simulink model "VSD_FD_codegen_V2"  (R2021b)
settings: Solver=FixedStepDiscrete  StartTime=0.0  StopTime=2  RelTol=1e-3  EnableMultiTasking=on
PreLoadFcn:
  | uz_setCodegenPaths
model workspace (MATLAB code in the model file):
  | cmdLim = Simulink.Parameter;
  | cmdLim.Value = 15;
  | cmdLim.Description = 'Limit for controlling the maximum surface command angle.';
  | cmdLim.Min = 0;
  | cmdLim.Max = 90;
  | cmdLim.DocUnits = 'deg';
  | 
  | dispGain = Simulink.Parameter;
  | dispGain.Value = 0.75;
  | dispGain.Description = 'Gain applied to the displacement error.';
  | dispGain.Min = 0;
  | dispGain.Max = [];
  | dispGain.DocUnits = 'deg/sec/deg';
  | 
  | dispLim = Simulink.Parameter;
  | dispLim.Value = 30;
  | dispLim.Description = 'Limit for controlling the maximum commanded angle.';
  | dispLim.Min = 0;
  | dispLim.Max = 180;
  | dispLim.DocUnits = 'deg';
  | 
  | intGain = Simulink.Parameter;
  | intGain.Value = 0.5;
  | intGain.Description = 'Gain applied to the integral error.';
  | intGain.Min = 0;
  | intGain.Max = [];
  | intGain.DocUnits = 'deg/sec/deg/sec';
  | 
  | intLim = Simulink.Parameter;
  | intLim.Value = 5;
  | intLim.Description = 'Limit for controlling the maximum commanded angle.';
  | intLim.Min = 0;
  | intLim.Max = 90;
  | intLim.DocUnits = 'deg';
  | 
  | rateGain = Simulink.Parameter;
  | rateGain.Value = 2;
  | rateGain.Description = 'Gain applied to the rate error.';
  | rateGain.Min = 0;
  | rateGain.Max = [];
  | rateGain.DocUnits = 'deg/deg/sec';
  | 
  | rateLim = Simulink.Parameter;
  | rateLim.Value = 6;
  | rateLim.Description = 'Limit for controlling the maximum commanded angle.';
  | rateLim.Min = 0;
  | rateLim.Max = 180;
  | rateLim.DocUnits = 'deg/sec';
  | 
  | hdgGain = Simulink.Parameter;
  | hdgGain.Value = 0.015;
undefined symbols (not defined in the file or in its folder): DiscIntNeverNeededParam, f_FD
libraries: simulink x203, dspstat3 x3, spsFirstOrderFilterLib x2
(part 2 of 2)

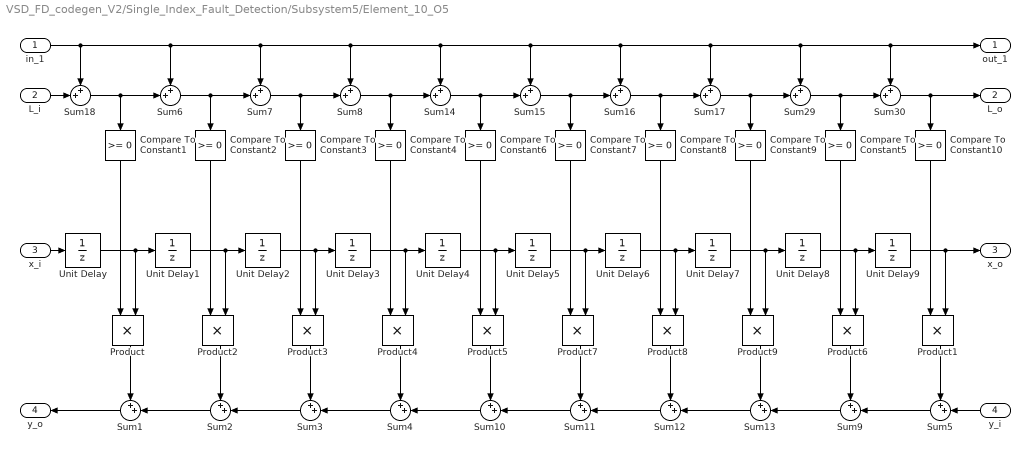
== system VSD_FD_codegen_V2/Single_Index_Fault_Detection/Subsystem5/Element_10_O5 ==
  in_1 : Inport
  L_i : Inport  Port=2
  x_i : Inport  Port=3
  y_i : Inport  Port=4
  Compare To Constant{1..10} (10 alike) : simulink/Logic and Bit Operations/Compare To Constant  relop=>=  const=0  OutDataTypeStr=boolean
  Product{,1..9} (10 alike) : Product
  Sum{1..18,29..30} (20 alike) : Sum  Inputs=++|
  Unit Delay{,1..9} (10 alike) : UnitDelay  SampleTime=-1  HasFrameUpgradeWarning=on
  out_1 : Outport
  L_o : Outport  Port=2
  x_o : Outport  Port=3
  y_o : Outport  Port=4
  wires:
  Sum2/1 -> Sum1/2
  Unit Delay4/1 -> Unit Delay5/1, Product5/2
  Unit Delay9/1 -> x_o/1, Product1/2
  Sum3/1 -> Sum2/2
  Sum6/1 -> Compare To Constant2/1, Sum7/2
  Sum15/1 -> Compare To Constant7/1, Sum16/2
  Sum9/1 -> Sum13/2
  Sum14/1 -> Sum15/2, Compare To Constant6/1
  Compare To Constant4/1 -> Product4/1
  Unit Delay7/1 -> Unit Delay8/1, Product9/2
  Unit Delay6/1 -> Unit Delay7/1, Product8/2
  Sum7/1 -> Compare To Constant3/1, Sum8/2
  Compare To Constant3/1 -> Product3/1
  Product8/1 -> Sum12/1
  Sum13/1 -> Sum12/2
  in_1/1 -> Sum18/1, Sum6/1, Sum7/1, Sum15/1, Sum16/1, out_1/1, Sum30/1, Sum29/1, Sum17/1, Sum14/1, Sum8/1
  Unit Delay8/1 -> Unit Delay9/1, Product6/2
  Product9/1 -> Sum13/1
  Sum11/1 -> Sum10/2
  Sum8/1 -> Compare To Constant4/1, Sum14/2
  Compare To Constant6/1 -> Product5/1
  Product7/1 -> Sum11/1
  Compare To Constant8/1 -> Product8/1
  Product/1 -> Sum1/1
  Unit Delay5/1 -> Unit Delay6/1, Product7/2
  Unit Delay/1 -> Unit Delay1/1, Product/2
  Unit Delay1/1 -> Unit Delay2/1, Product2/2
  Compare To Constant5/1 -> Product6/1
  Sum10/1 -> Sum4/2
  Sum1/1 -> y_o/1
  Compare To Constant2/1 -> Product2/1
  Sum16/1 -> Compare To Constant8/1, Sum17/2
  Compare To Constant1/1 -> Product/1
  Sum4/1 -> Sum3/2
  Sum17/1 -> Sum29/2, Compare To Constant9/1
  Unit Delay3/1 -> Unit Delay4/1, Product4/2
  Product5/1 -> Sum10/1
  Product6/1 -> Sum9/1
  Sum12/1 -> Sum11/2
  Sum29/1 -> Sum30/2, Compare To Constant5/1
  Sum30/1 -> L_o/1, Compare To Constant10/1
  Product4/1 -> Sum4/1
  Product2/1 -> Sum2/1
  Unit Delay2/1 -> Unit Delay3/1, Product3/2
  Compare To Constant9/1 -> Product9/1
  Product3/1 -> Sum3/1
  x_i/1 -> Unit Delay/1
  Compare To Constant7/1 -> Product7/1
  Compare To Constant10/1 -> Product1/1
  Product1/1 -> Sum5/1
  y_i/1 -> Sum5/2
  Sum5/1 -> Sum9/2
  L_i/1 -> Sum18/2
  Sum18/1 -> Compare To Constant1/1, Sum6/2

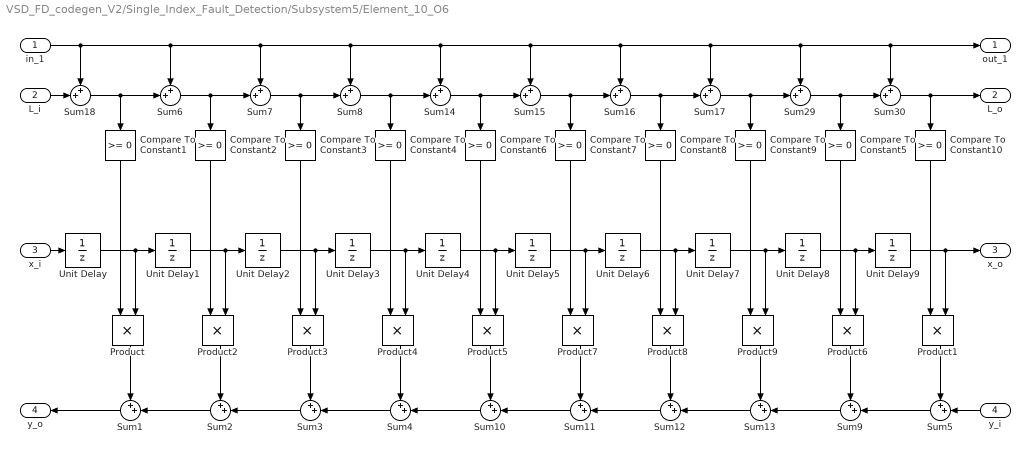
== system VSD_FD_codegen_V2/Single_Index_Fault_Detection/Subsystem5/Element_10_O6 ==
  in_1 : Inport
  L_i : Inport  Port=2
  x_i : Inport  Port=3
  y_i : Inport  Port=4
  Compare To Constant{1..10} (10 alike) : simulink/Logic and Bit Operations/Compare To Constant  relop=>=  const=0  OutDataTypeStr=boolean
  Product{,1..9} (10 alike) : Product
  Sum{1..18,29..30} (20 alike) : Sum  Inputs=++|
  Unit Delay{,1..9} (10 alike) : UnitDelay  SampleTime=-1  HasFrameUpgradeWarning=on
  out_1 : Outport
  L_o : Outport  Port=2
  x_o : Outport  Port=3
  y_o : Outport  Port=4
  wires:
  Sum2/1 -> Sum1/2
  Unit Delay4/1 -> Unit Delay5/1, Product5/2
  Unit Delay9/1 -> x_o/1, Product1/2
  Sum3/1 -> Sum2/2
  Sum6/1 -> Compare To Constant2/1, Sum7/2
  Sum15/1 -> Compare To Constant7/1, Sum16/2
  Sum9/1 -> Sum13/2
  Sum14/1 -> Sum15/2, Compare To Constant6/1
  Compare To Constant4/1 -> Product4/1
  Unit Delay7/1 -> Unit Delay8/1, Product9/2
  Unit Delay6/1 -> Unit Delay7/1, Product8/2
  Sum7/1 -> Compare To Constant3/1, Sum8/2
  Compare To Constant3/1 -> Product3/1
  Product8/1 -> Sum12/1
  Sum13/1 -> Sum12/2
  in_1/1 -> Sum18/1, Sum6/1, Sum7/1, Sum15/1, Sum16/1, out_1/1, Sum30/1, Sum29/1, Sum17/1, Sum14/1, Sum8/1
  Unit Delay8/1 -> Unit Delay9/1, Product6/2
  Product9/1 -> Sum13/1
  Sum11/1 -> Sum10/2
  Sum8/1 -> Compare To Constant4/1, Sum14/2
  Compare To Constant6/1 -> Product5/1
  Product7/1 -> Sum11/1
  Compare To Constant8/1 -> Product8/1
  Product/1 -> Sum1/1
  Unit Delay5/1 -> Unit Delay6/1, Product7/2
  Unit Delay/1 -> Unit Delay1/1, Product/2
  Unit Delay1/1 -> Unit Delay2/1, Product2/2
  Compare To Constant5/1 -> Product6/1
  Sum10/1 -> Sum4/2
  Sum1/1 -> y_o/1
  Compare To Constant2/1 -> Product2/1
  Sum16/1 -> Compare To Constant8/1, Sum17/2
  Compare To Constant1/1 -> Product/1
  Sum4/1 -> Sum3/2
  Sum17/1 -> Sum29/2, Compare To Constant9/1
  Unit Delay3/1 -> Unit Delay4/1, Product4/2
  Product5/1 -> Sum10/1
  Product6/1 -> Sum9/1
  Sum12/1 -> Sum11/2
  Sum29/1 -> Sum30/2, Compare To Constant5/1
  Sum30/1 -> L_o/1, Compare To Constant10/1
  Product4/1 -> Sum4/1
  Product2/1 -> Sum2/1
  Unit Delay2/1 -> Unit Delay3/1, Product3/2
  Compare To Constant9/1 -> Product9/1
  Product3/1 -> Sum3/1
  x_i/1 -> Unit Delay/1
  Compare To Constant7/1 -> Product7/1
  Compare To Constant10/1 -> Product1/1
  Product1/1 -> Sum5/1
  y_i/1 -> Sum5/2
  Sum5/1 -> Sum9/2
  L_i/1 -> Sum18/2
  Sum18/1 -> Compare To Constant1/1, Sum6/2

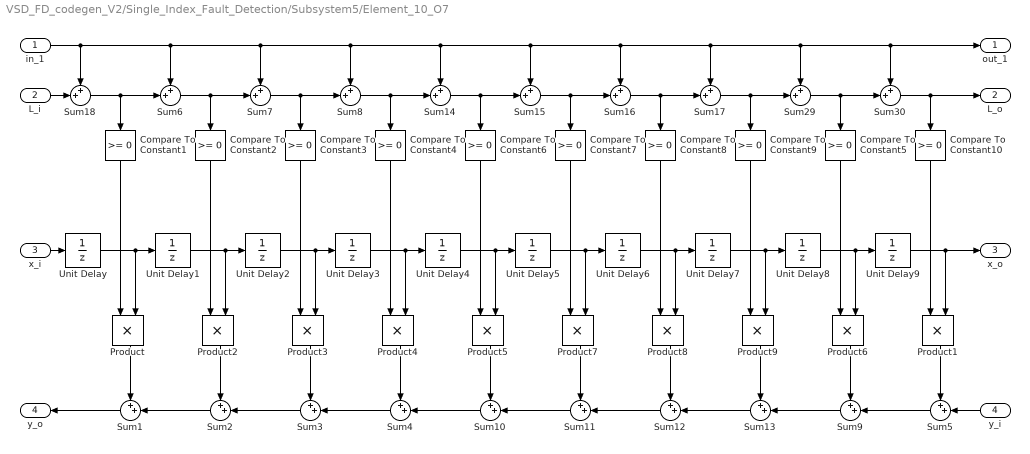
== system VSD_FD_codegen_V2/Single_Index_Fault_Detection/Subsystem5/Element_10_O7 ==
  in_1 : Inport
  L_i : Inport  Port=2
  x_i : Inport  Port=3
  y_i : Inport  Port=4
  Compare To Constant{1..10} (10 alike) : simulink/Logic and Bit Operations/Compare To Constant  relop=>=  const=0  OutDataTypeStr=boolean
  Product{,1..9} (10 alike) : Product
  Sum{1..18,29..30} (20 alike) : Sum  Inputs=++|
  Unit Delay{,1..9} (10 alike) : UnitDelay  SampleTime=-1  HasFrameUpgradeWarning=on
  out_1 : Outport
  L_o : Outport  Port=2
  x_o : Outport  Port=3
  y_o : Outport  Port=4
  wires:
  Sum2/1 -> Sum1/2
  Unit Delay4/1 -> Unit Delay5/1, Product5/2
  Unit Delay9/1 -> x_o/1, Product1/2
  Sum3/1 -> Sum2/2
  Sum6/1 -> Compare To Constant2/1, Sum7/2
  Sum15/1 -> Compare To Constant7/1, Sum16/2
  Sum9/1 -> Sum13/2
  Sum14/1 -> Sum15/2, Compare To Constant6/1
  Compare To Constant4/1 -> Product4/1
  Unit Delay7/1 -> Unit Delay8/1, Product9/2
  Unit Delay6/1 -> Unit Delay7/1, Product8/2
  Sum7/1 -> Compare To Constant3/1, Sum8/2
  Compare To Constant3/1 -> Product3/1
  Product8/1 -> Sum12/1
  Sum13/1 -> Sum12/2
  in_1/1 -> Sum18/1, Sum6/1, Sum7/1, Sum15/1, Sum16/1, out_1/1, Sum30/1, Sum29/1, Sum17/1, Sum14/1, Sum8/1
  Unit Delay8/1 -> Unit Delay9/1, Product6/2
  Product9/1 -> Sum13/1
  Sum11/1 -> Sum10/2
  Sum8/1 -> Compare To Constant4/1, Sum14/2
  Compare To Constant6/1 -> Product5/1
  Product7/1 -> Sum11/1
  Compare To Constant8/1 -> Product8/1
  Product/1 -> Sum1/1
  Unit Delay5/1 -> Unit Delay6/1, Product7/2
  Unit Delay/1 -> Unit Delay1/1, Product/2
  Unit Delay1/1 -> Unit Delay2/1, Product2/2
  Compare To Constant5/1 -> Product6/1
  Sum10/1 -> Sum4/2
  Sum1/1 -> y_o/1
  Compare To Constant2/1 -> Product2/1
  Sum16/1 -> Compare To Constant8/1, Sum17/2
  Compare To Constant1/1 -> Product/1
  Sum4/1 -> Sum3/2
  Sum17/1 -> Sum29/2, Compare To Constant9/1
  Unit Delay3/1 -> Unit Delay4/1, Product4/2
  Product5/1 -> Sum10/1
  Product6/1 -> Sum9/1
  Sum12/1 -> Sum11/2
  Sum29/1 -> Sum30/2, Compare To Constant5/1
  Sum30/1 -> L_o/1, Compare To Constant10/1
  Product4/1 -> Sum4/1
  Product2/1 -> Sum2/1
  Unit Delay2/1 -> Unit Delay3/1, Product3/2
  Compare To Constant9/1 -> Product9/1
  Product3/1 -> Sum3/1
  x_i/1 -> Unit Delay/1
  Compare To Constant7/1 -> Product7/1
  Compare To Constant10/1 -> Product1/1
  Product1/1 -> Sum5/1
  y_i/1 -> Sum5/2
  Sum5/1 -> Sum9/2
  L_i/1 -> Sum18/2
  Sum18/1 -> Compare To Constant1/1, Sum6/2

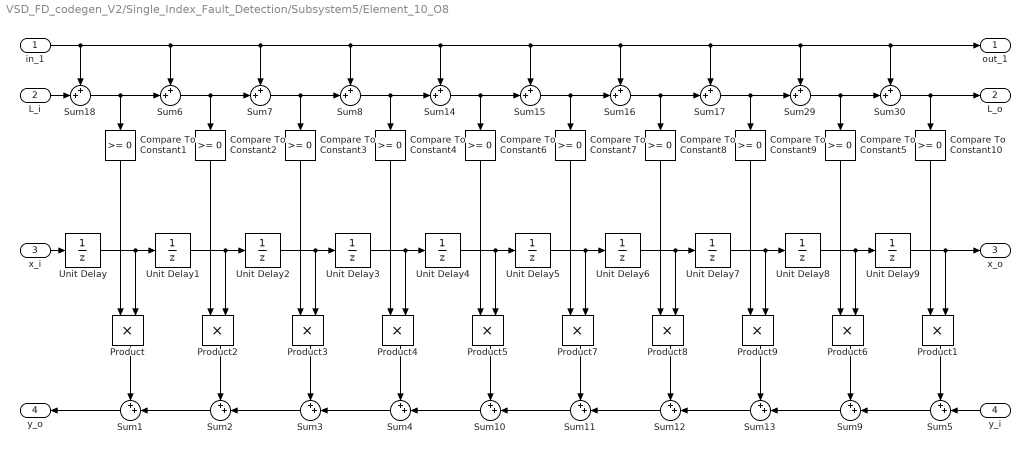
== system VSD_FD_codegen_V2/Single_Index_Fault_Detection/Subsystem5/Element_10_O8 ==
  in_1 : Inport
  L_i : Inport  Port=2
  x_i : Inport  Port=3
  y_i : Inport  Port=4
  Compare To Constant{1..10} (10 alike) : simulink/Logic and Bit Operations/Compare To Constant  relop=>=  const=0  OutDataTypeStr=boolean
  Product{,1..9} (10 alike) : Product
  Sum{1..18,29..30} (20 alike) : Sum  Inputs=++|
  Unit Delay{,1..9} (10 alike) : UnitDelay  SampleTime=-1  HasFrameUpgradeWarning=on
  out_1 : Outport
  L_o : Outport  Port=2
  x_o : Outport  Port=3
  y_o : Outport  Port=4
  wires:
  Sum2/1 -> Sum1/2
  Unit Delay4/1 -> Unit Delay5/1, Product5/2
  Unit Delay9/1 -> x_o/1, Product1/2
  Sum3/1 -> Sum2/2
  Sum6/1 -> Compare To Constant2/1, Sum7/2
  Sum15/1 -> Compare To Constant7/1, Sum16/2
  Sum9/1 -> Sum13/2
  Sum14/1 -> Sum15/2, Compare To Constant6/1
  Compare To Constant4/1 -> Product4/1
  Unit Delay7/1 -> Unit Delay8/1, Product9/2
  Unit Delay6/1 -> Unit Delay7/1, Product8/2
  Sum7/1 -> Compare To Constant3/1, Sum8/2
  Compare To Constant3/1 -> Product3/1
  Product8/1 -> Sum12/1
  Sum13/1 -> Sum12/2
  in_1/1 -> Sum18/1, Sum6/1, Sum7/1, Sum15/1, Sum16/1, out_1/1, Sum30/1, Sum29/1, Sum17/1, Sum14/1, Sum8/1
  Unit Delay8/1 -> Unit Delay9/1, Product6/2
  Product9/1 -> Sum13/1
  Sum11/1 -> Sum10/2
  Sum8/1 -> Compare To Constant4/1, Sum14/2
  Compare To Constant6/1 -> Product5/1
  Product7/1 -> Sum11/1
  Compare To Constant8/1 -> Product8/1
  Product/1 -> Sum1/1
  Unit Delay5/1 -> Unit Delay6/1, Product7/2
  Unit Delay/1 -> Unit Delay1/1, Product/2
  Unit Delay1/1 -> Unit Delay2/1, Product2/2
  Compare To Constant5/1 -> Product6/1
  Sum10/1 -> Sum4/2
  Sum1/1 -> y_o/1
  Compare To Constant2/1 -> Product2/1
  Sum16/1 -> Compare To Constant8/1, Sum17/2
  Compare To Constant1/1 -> Product/1
  Sum4/1 -> Sum3/2
  Sum17/1 -> Sum29/2, Compare To Constant9/1
  Unit Delay3/1 -> Unit Delay4/1, Product4/2
  Product5/1 -> Sum10/1
  Product6/1 -> Sum9/1
  Sum12/1 -> Sum11/2
  Sum29/1 -> Sum30/2, Compare To Constant5/1
  Sum30/1 -> L_o/1, Compare To Constant10/1
  Product4/1 -> Sum4/1
  Product2/1 -> Sum2/1
  Unit Delay2/1 -> Unit Delay3/1, Product3/2
  Compare To Constant9/1 -> Product9/1
  Product3/1 -> Sum3/1
  x_i/1 -> Unit Delay/1
  Compare To Constant7/1 -> Product7/1
  Compare To Constant10/1 -> Product1/1
  Product1/1 -> Sum5/1
  y_i/1 -> Sum5/2
  Sum5/1 -> Sum9/2
  L_i/1 -> Sum18/2
  Sum18/1 -> Compare To Constant1/1, Sum6/2

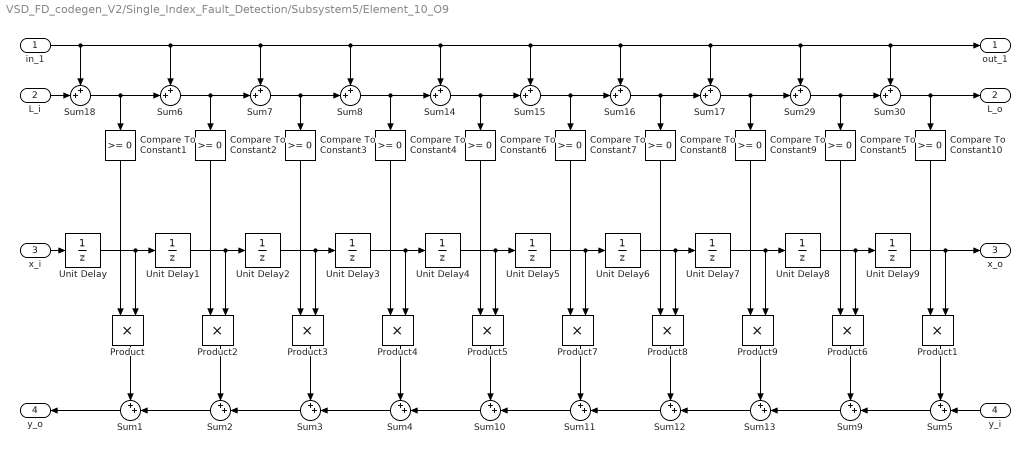
== system VSD_FD_codegen_V2/Single_Index_Fault_Detection/Subsystem5/Element_10_O9 ==
  in_1 : Inport
  L_i : Inport  Port=2
  x_i : Inport  Port=3
  y_i : Inport  Port=4
  Compare To Constant{1..10} (10 alike) : simulink/Logic and Bit Operations/Compare To Constant  relop=>=  const=0  OutDataTypeStr=boolean
  Product{,1..9} (10 alike) : Product
  Sum{1..18,29..30} (20 alike) : Sum  Inputs=++|
  Unit Delay{,1..9} (10 alike) : UnitDelay  SampleTime=-1  HasFrameUpgradeWarning=on
  out_1 : Outport
  L_o : Outport  Port=2
  x_o : Outport  Port=3
  y_o : Outport  Port=4
  wires:
  Sum2/1 -> Sum1/2
  Unit Delay4/1 -> Unit Delay5/1, Product5/2
  Unit Delay9/1 -> x_o/1, Product1/2
  Sum3/1 -> Sum2/2
  Sum6/1 -> Compare To Constant2/1, Sum7/2
  Sum15/1 -> Compare To Constant7/1, Sum16/2
  Sum9/1 -> Sum13/2
  Sum14/1 -> Sum15/2, Compare To Constant6/1
  Compare To Constant4/1 -> Product4/1
  Unit Delay7/1 -> Unit Delay8/1, Product9/2
  Unit Delay6/1 -> Unit Delay7/1, Product8/2
  Sum7/1 -> Compare To Constant3/1, Sum8/2
  Compare To Constant3/1 -> Product3/1
  Product8/1 -> Sum12/1
  Sum13/1 -> Sum12/2
  in_1/1 -> Sum18/1, Sum6/1, Sum7/1, Sum15/1, Sum16/1, out_1/1, Sum30/1, Sum29/1, Sum17/1, Sum14/1, Sum8/1
  Unit Delay8/1 -> Unit Delay9/1, Product6/2
  Product9/1 -> Sum13/1
  Sum11/1 -> Sum10/2
  Sum8/1 -> Compare To Constant4/1, Sum14/2
  Compare To Constant6/1 -> Product5/1
  Product7/1 -> Sum11/1
  Compare To Constant8/1 -> Product8/1
  Product/1 -> Sum1/1
  Unit Delay5/1 -> Unit Delay6/1, Product7/2
  Unit Delay/1 -> Unit Delay1/1, Product/2
  Unit Delay1/1 -> Unit Delay2/1, Product2/2
  Compare To Constant5/1 -> Product6/1
  Sum10/1 -> Sum4/2
  Sum1/1 -> y_o/1
  Compare To Constant2/1 -> Product2/1
  Sum16/1 -> Compare To Constant8/1, Sum17/2
  Compare To Constant1/1 -> Product/1
  Sum4/1 -> Sum3/2
  Sum17/1 -> Sum29/2, Compare To Constant9/1
  Unit Delay3/1 -> Unit Delay4/1, Product4/2
  Product5/1 -> Sum10/1
  Product6/1 -> Sum9/1
  Sum12/1 -> Sum11/2
  Sum29/1 -> Sum30/2, Compare To Constant5/1
  Sum30/1 -> L_o/1, Compare To Constant10/1
  Product4/1 -> Sum4/1
  Product2/1 -> Sum2/1
  Unit Delay2/1 -> Unit Delay3/1, Product3/2
  Compare To Constant9/1 -> Product9/1
  Product3/1 -> Sum3/1
  x_i/1 -> Unit Delay/1
  Compare To Constant7/1 -> Product7/1
  Compare To Constant10/1 -> Product1/1
  Product1/1 -> Sum5/1
  y_i/1 -> Sum5/2
  Sum5/1 -> Sum9/2
  L_i/1 -> Sum18/2
  Sum18/1 -> Compare To Constant1/1, Sum6/2

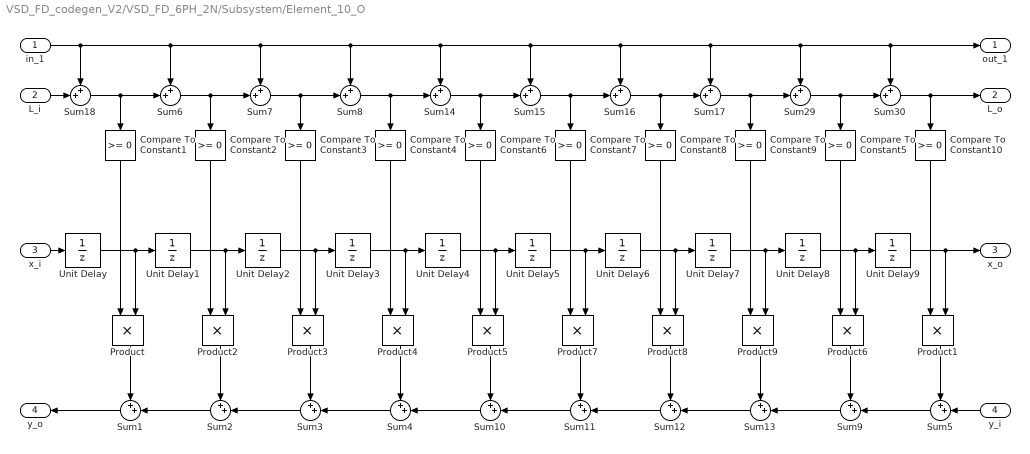
== system VSD_FD_codegen_V2/VSD_FD_6PH_2N/Subsystem/Element_10_O ==
  in_1 : Inport
  L_i : Inport  Port=2
  x_i : Inport  Port=3
  y_i : Inport  Port=4
  Compare To Constant{1..10} (10 alike) : simulink/Logic and Bit Operations/Compare To Constant  relop=>=  const=0  OutDataTypeStr=boolean
  Product{,1..9} (10 alike) : Product
  Sum{1..18,29..30} (20 alike) : Sum  Inputs=++|
  Unit Delay{,1..9} (10 alike) : UnitDelay  SampleTime=-1  HasFrameUpgradeWarning=on
  out_1 : Outport
  L_o : Outport  Port=2
  x_o : Outport  Port=3
  y_o : Outport  Port=4
  wires:
  Sum2/1 -> Sum1/2
  Unit Delay4/1 -> Unit Delay5/1, Product5/2
  Unit Delay9/1 -> x_o/1, Product1/2
  Sum3/1 -> Sum2/2
  Sum6/1 -> Compare To Constant2/1, Sum7/2
  Sum15/1 -> Compare To Constant7/1, Sum16/2
  Sum9/1 -> Sum13/2
  Sum14/1 -> Sum15/2, Compare To Constant6/1
  Compare To Constant4/1 -> Product4/1
  Unit Delay7/1 -> Unit Delay8/1, Product9/2
  Unit Delay6/1 -> Unit Delay7/1, Product8/2
  Sum7/1 -> Compare To Constant3/1, Sum8/2
  Compare To Constant3/1 -> Product3/1
  Product8/1 -> Sum12/1
  Sum13/1 -> Sum12/2
  in_1/1 -> Sum18/1, Sum6/1, Sum7/1, Sum15/1, Sum16/1, out_1/1, Sum30/1, Sum29/1, Sum17/1, Sum14/1, Sum8/1
  Unit Delay8/1 -> Unit Delay9/1, Product6/2
  Product9/1 -> Sum13/1
  Sum11/1 -> Sum10/2
  Sum8/1 -> Compare To Constant4/1, Sum14/2
  Compare To Constant6/1 -> Product5/1
  Product7/1 -> Sum11/1
  Compare To Constant8/1 -> Product8/1
  Product/1 -> Sum1/1
  Unit Delay5/1 -> Unit Delay6/1, Product7/2
  Unit Delay/1 -> Unit Delay1/1, Product/2
  Unit Delay1/1 -> Unit Delay2/1, Product2/2
  Compare To Constant5/1 -> Product6/1
  Sum10/1 -> Sum4/2
  Sum1/1 -> y_o/1
  Compare To Constant2/1 -> Product2/1
  Sum16/1 -> Compare To Constant8/1, Sum17/2
  Compare To Constant1/1 -> Product/1
  Sum4/1 -> Sum3/2
  Sum17/1 -> Sum29/2, Compare To Constant9/1
  Unit Delay3/1 -> Unit Delay4/1, Product4/2
  Product5/1 -> Sum10/1
  Product6/1 -> Sum9/1
  Sum12/1 -> Sum11/2
  Sum29/1 -> Sum30/2, Compare To Constant5/1
  Sum30/1 -> L_o/1, Compare To Constant10/1
  Product4/1 -> Sum4/1
  Product2/1 -> Sum2/1
  Unit Delay2/1 -> Unit Delay3/1, Product3/2
  Compare To Constant9/1 -> Product9/1
  Product3/1 -> Sum3/1
  x_i/1 -> Unit Delay/1
  Compare To Constant7/1 -> Product7/1
  Compare To Constant10/1 -> Product1/1
  Product1/1 -> Sum5/1
  y_i/1 -> Sum5/2
  Sum5/1 -> Sum9/2
  L_i/1 -> Sum18/2
  Sum18/1 -> Compare To Constant1/1, Sum6/2

== system VSD_FD_codegen_V2/VSD_FD_6PH_2N/Subsystem/Element_10_O1 ==
  in_1 : Inport
  L_i : Inport  Port=2
  x_i : Inport  Port=3
  y_i : Inport  Port=4
  Compare To Constant{1..10} (10 alike) : simulink/Logic and Bit Operations/Compare To Constant  relop=>=  const=0  OutDataTypeStr=boolean
  Product{,1..9} (10 alike) : Product
  Sum{1..18,29..30} (20 alike) : Sum  Inputs=++|
  Unit Delay{,1..9} (10 alike) : UnitDelay  SampleTime=-1  HasFrameUpgradeWarning=on
  out_1 : Outport
  L_o : Outport  Port=2
  x_o : Outport  Port=3
  y_o : Outport  Port=4
  wires:
  Sum2/1 -> Sum1/2
  Unit Delay4/1 -> Unit Delay5/1, Product5/2
  Unit Delay9/1 -> x_o/1, Product1/2
  Sum3/1 -> Sum2/2
  Sum6/1 -> Compare To Constant2/1, Sum7/2
  Sum15/1 -> Compare To Constant7/1, Sum16/2
  Sum9/1 -> Sum13/2
  Sum14/1 -> Sum15/2, Compare To Constant6/1
  Compare To Constant4/1 -> Product4/1
  Unit Delay7/1 -> Unit Delay8/1, Product9/2
  Unit Delay6/1 -> Unit Delay7/1, Product8/2
  Sum7/1 -> Compare To Constant3/1, Sum8/2
  Compare To Constant3/1 -> Product3/1
  Product8/1 -> Sum12/1
  Sum13/1 -> Sum12/2
  in_1/1 -> Sum18/1, Sum6/1, Sum7/1, Sum15/1, Sum16/1, out_1/1, Sum30/1, Sum29/1, Sum17/1, Sum14/1, Sum8/1
  Unit Delay8/1 -> Unit Delay9/1, Product6/2
  Product9/1 -> Sum13/1
  Sum11/1 -> Sum10/2
  Sum8/1 -> Compare To Constant4/1, Sum14/2
  Compare To Constant6/1 -> Product5/1
  Product7/1 -> Sum11/1
  Compare To Constant8/1 -> Product8/1
  Product/1 -> Sum1/1
  Unit Delay5/1 -> Unit Delay6/1, Product7/2
  Unit Delay/1 -> Unit Delay1/1, Product/2
  Unit Delay1/1 -> Unit Delay2/1, Product2/2
  Compare To Constant5/1 -> Product6/1
  Sum10/1 -> Sum4/2
  Sum1/1 -> y_o/1
  Compare To Constant2/1 -> Product2/1
  Sum16/1 -> Compare To Constant8/1, Sum17/2
  Compare To Constant1/1 -> Product/1
  Sum4/1 -> Sum3/2
  Sum17/1 -> Sum29/2, Compare To Constant9/1
  Unit Delay3/1 -> Unit Delay4/1, Product4/2
  Product5/1 -> Sum10/1
  Product6/1 -> Sum9/1
  Sum12/1 -> Sum11/2
  Sum29/1 -> Sum30/2, Compare To Constant5/1
  Sum30/1 -> L_o/1, Compare To Constant10/1
  Product4/1 -> Sum4/1
  Product2/1 -> Sum2/1
  Unit Delay2/1 -> Unit Delay3/1, Product3/2
  Compare To Constant9/1 -> Product9/1
  Product3/1 -> Sum3/1
  x_i/1 -> Unit Delay/1
  Compare To Constant7/1 -> Product7/1
  Compare To Constant10/1 -> Product1/1
  Product1/1 -> Sum5/1
  y_i/1 -> Sum5/2
  Sum5/1 -> Sum9/2
  L_i/1 -> Sum18/2
  Sum18/1 -> Compare To Constant1/1, Sum6/2

== system VSD_FD_codegen_V2/VSD_FD_6PH_2N/Subsystem/Element_10_O2 ==
  in_1 : Inport
  L_i : Inport  Port=2
  x_i : Inport  Port=3
  y_i : Inport  Port=4
  Compare To Constant{1..10} (10 alike) : simulink/Logic and Bit Operations/Compare To Constant  relop=>=  const=0  OutDataTypeStr=boolean
  Product{,1..9} (10 alike) : Product
  Sum{1..18,29..30} (20 alike) : Sum  Inputs=++|
  Unit Delay{,1..9} (10 alike) : UnitDelay  SampleTime=-1  HasFrameUpgradeWarning=on
  out_1 : Outport
  L_o : Outport  Port=2
  x_o : Outport  Port=3
  y_o : Outport  Port=4
  wires:
  Sum2/1 -> Sum1/2
  Unit Delay4/1 -> Unit Delay5/1, Product5/2
  Unit Delay9/1 -> x_o/1, Product1/2
  Sum3/1 -> Sum2/2
  Sum6/1 -> Compare To Constant2/1, Sum7/2
  Sum15/1 -> Compare To Constant7/1, Sum16/2
  Sum9/1 -> Sum13/2
  Sum14/1 -> Sum15/2, Compare To Constant6/1
  Compare To Constant4/1 -> Product4/1
  Unit Delay7/1 -> Unit Delay8/1, Product9/2
  Unit Delay6/1 -> Unit Delay7/1, Product8/2
  Sum7/1 -> Compare To Constant3/1, Sum8/2
  Compare To Constant3/1 -> Product3/1
  Product8/1 -> Sum12/1
  Sum13/1 -> Sum12/2
  in_1/1 -> Sum18/1, Sum6/1, Sum7/1, Sum15/1, Sum16/1, out_1/1, Sum30/1, Sum29/1, Sum17/1, Sum14/1, Sum8/1
  Unit Delay8/1 -> Unit Delay9/1, Product6/2
  Product9/1 -> Sum13/1
  Sum11/1 -> Sum10/2
  Sum8/1 -> Compare To Constant4/1, Sum14/2
  Compare To Constant6/1 -> Product5/1
  Product7/1 -> Sum11/1
  Compare To Constant8/1 -> Product8/1
  Product/1 -> Sum1/1
  Unit Delay5/1 -> Unit Delay6/1, Product7/2
  Unit Delay/1 -> Unit Delay1/1, Product/2
  Unit Delay1/1 -> Unit Delay2/1, Product2/2
  Compare To Constant5/1 -> Product6/1
  Sum10/1 -> Sum4/2
  Sum1/1 -> y_o/1
  Compare To Constant2/1 -> Product2/1
  Sum16/1 -> Compare To Constant8/1, Sum17/2
  Compare To Constant1/1 -> Product/1
  Sum4/1 -> Sum3/2
  Sum17/1 -> Sum29/2, Compare To Constant9/1
  Unit Delay3/1 -> Unit Delay4/1, Product4/2
  Product5/1 -> Sum10/1
  Product6/1 -> Sum9/1
  Sum12/1 -> Sum11/2
  Sum29/1 -> Sum30/2, Compare To Constant5/1
  Sum30/1 -> L_o/1, Compare To Constant10/1
  Product4/1 -> Sum4/1
  Product2/1 -> Sum2/1
  Unit Delay2/1 -> Unit Delay3/1, Product3/2
  Compare To Constant9/1 -> Product9/1
  Product3/1 -> Sum3/1
  x_i/1 -> Unit Delay/1
  Compare To Constant7/1 -> Product7/1
  Compare To Constant10/1 -> Product1/1
  Product1/1 -> Sum5/1
  y_i/1 -> Sum5/2
  Sum5/1 -> Sum9/2
  L_i/1 -> Sum18/2
  Sum18/1 -> Compare To Constant1/1, Sum6/2

== system VSD_FD_codegen_V2/VSD_FD_6PH_2N/Subsystem/Element_10_O3 ==
  in_1 : Inport
  L_i : Inport  Port=2
  x_i : Inport  Port=3
  y_i : Inport  Port=4
  Compare To Constant{1..10} (10 alike) : simulink/Logic and Bit Operations/Compare To Constant  relop=>=  const=0  OutDataTypeStr=boolean
  Product{,1..9} (10 alike) : Product
  Sum{1..18,29..30} (20 alike) : Sum  Inputs=++|
  Unit Delay{,1..9} (10 alike) : UnitDelay  SampleTime=-1  HasFrameUpgradeWarning=on
  out_1 : Outport
  L_o : Outport  Port=2
  x_o : Outport  Port=3
  y_o : Outport  Port=4
  wires:
  Sum2/1 -> Sum1/2
  Unit Delay4/1 -> Unit Delay5/1, Product5/2
  Unit Delay9/1 -> x_o/1, Product1/2
  Sum3/1 -> Sum2/2
  Sum6/1 -> Compare To Constant2/1, Sum7/2
  Sum15/1 -> Compare To Constant7/1, Sum16/2
  Sum9/1 -> Sum13/2
  Sum14/1 -> Sum15/2, Compare To Constant6/1
  Compare To Constant4/1 -> Product4/1
  Unit Delay7/1 -> Unit Delay8/1, Product9/2
  Unit Delay6/1 -> Unit Delay7/1, Product8/2
  Sum7/1 -> Compare To Constant3/1, Sum8/2
  Compare To Constant3/1 -> Product3/1
  Product8/1 -> Sum12/1
  Sum13/1 -> Sum12/2
  in_1/1 -> Sum18/1, Sum6/1, Sum7/1, Sum15/1, Sum16/1, out_1/1, Sum30/1, Sum29/1, Sum17/1, Sum14/1, Sum8/1
  Unit Delay8/1 -> Unit Delay9/1, Product6/2
  Product9/1 -> Sum13/1
  Sum11/1 -> Sum10/2
  Sum8/1 -> Compare To Constant4/1, Sum14/2
  Compare To Constant6/1 -> Product5/1
  Product7/1 -> Sum11/1
  Compare To Constant8/1 -> Product8/1
  Product/1 -> Sum1/1
  Unit Delay5/1 -> Unit Delay6/1, Product7/2
  Unit Delay/1 -> Unit Delay1/1, Product/2
  Unit Delay1/1 -> Unit Delay2/1, Product2/2
  Compare To Constant5/1 -> Product6/1
  Sum10/1 -> Sum4/2
  Sum1/1 -> y_o/1
  Compare To Constant2/1 -> Product2/1
  Sum16/1 -> Compare To Constant8/1, Sum17/2
  Compare To Constant1/1 -> Product/1
  Sum4/1 -> Sum3/2
  Sum17/1 -> Sum29/2, Compare To Constant9/1
  Unit Delay3/1 -> Unit Delay4/1, Product4/2
  Product5/1 -> Sum10/1
  Product6/1 -> Sum9/1
  Sum12/1 -> Sum11/2
  Sum29/1 -> Sum30/2, Compare To Constant5/1
  Sum30/1 -> L_o/1, Compare To Constant10/1
  Product4/1 -> Sum4/1
  Product2/1 -> Sum2/1
  Unit Delay2/1 -> Unit Delay3/1, Product3/2
  Compare To Constant9/1 -> Product9/1
  Product3/1 -> Sum3/1
  x_i/1 -> Unit Delay/1
  Compare To Constant7/1 -> Product7/1
  Compare To Constant10/1 -> Product1/1
  Product1/1 -> Sum5/1
  y_i/1 -> Sum5/2
  Sum5/1 -> Sum9/2
  L_i/1 -> Sum18/2
  Sum18/1 -> Compare To Constant1/1, Sum6/2

== system VSD_FD_codegen_V2/VSD_FD_6PH_2N/Subsystem/Element_10_O4 ==
  in_1 : Inport
  L_i : Inport  Port=2
  x_i : Inport  Port=3
  y_i : Inport  Port=4
  Compare To Constant{1..10} (10 alike) : simulink/Logic and Bit Operations/Compare To Constant  relop=>=  const=0  OutDataTypeStr=boolean
  Product{,1..9} (10 alike) : Product
  Sum{1..18,29..30} (20 alike) : Sum  Inputs=++|
  Unit Delay{,1..9} (10 alike) : UnitDelay  SampleTime=-1  HasFrameUpgradeWarning=on
  out_1 : Outport
  L_o : Outport  Port=2
  x_o : Outport  Port=3
  y_o : Outport  Port=4
  wires:
  Sum2/1 -> Sum1/2
  Unit Delay4/1 -> Unit Delay5/1, Product5/2
  Unit Delay9/1 -> x_o/1, Product1/2
  Sum3/1 -> Sum2/2
  Sum6/1 -> Compare To Constant2/1, Sum7/2
  Sum15/1 -> Compare To Constant7/1, Sum16/2
  Sum9/1 -> Sum13/2
  Sum14/1 -> Sum15/2, Compare To Constant6/1
  Compare To Constant4/1 -> Product4/1
  Unit Delay7/1 -> Unit Delay8/1, Product9/2
  Unit Delay6/1 -> Unit Delay7/1, Product8/2
  Sum7/1 -> Compare To Constant3/1, Sum8/2
  Compare To Constant3/1 -> Product3/1
  Product8/1 -> Sum12/1
  Sum13/1 -> Sum12/2
  in_1/1 -> Sum18/1, Sum6/1, Sum7/1, Sum15/1, Sum16/1, out_1/1, Sum30/1, Sum29/1, Sum17/1, Sum14/1, Sum8/1
  Unit Delay8/1 -> Unit Delay9/1, Product6/2
  Product9/1 -> Sum13/1
  Sum11/1 -> Sum10/2
  Sum8/1 -> Compare To Constant4/1, Sum14/2
  Compare To Constant6/1 -> Product5/1
  Product7/1 -> Sum11/1
  Compare To Constant8/1 -> Product8/1
  Product/1 -> Sum1/1
  Unit Delay5/1 -> Unit Delay6/1, Product7/2
  Unit Delay/1 -> Unit Delay1/1, Product/2
  Unit Delay1/1 -> Unit Delay2/1, Product2/2
  Compare To Constant5/1 -> Product6/1
  Sum10/1 -> Sum4/2
  Sum1/1 -> y_o/1
  Compare To Constant2/1 -> Product2/1
  Sum16/1 -> Compare To Constant8/1, Sum17/2
  Compare To Constant1/1 -> Product/1
  Sum4/1 -> Sum3/2
  Sum17/1 -> Sum29/2, Compare To Constant9/1
  Unit Delay3/1 -> Unit Delay4/1, Product4/2
  Product5/1 -> Sum10/1
  Product6/1 -> Sum9/1
  Sum12/1 -> Sum11/2
  Sum29/1 -> Sum30/2, Compare To Constant5/1
  Sum30/1 -> L_o/1, Compare To Constant10/1
  Product4/1 -> Sum4/1
  Product2/1 -> Sum2/1
  Unit Delay2/1 -> Unit Delay3/1, Product3/2
  Compare To Constant9/1 -> Product9/1
  Product3/1 -> Sum3/1
  x_i/1 -> Unit Delay/1
  Compare To Constant7/1 -> Product7/1
  Compare To Constant10/1 -> Product1/1
  Product1/1 -> Sum5/1
  y_i/1 -> Sum5/2
  Sum5/1 -> Sum9/2
  L_i/1 -> Sum18/2
  Sum18/1 -> Compare To Constant1/1, Sum6/2

== system VSD_FD_codegen_V2/VSD_FD_6PH_2N/Subsystem/Element_10_O5 ==
  in_1 : Inport
  L_i : Inport  Port=2
  x_i : Inport  Port=3
  y_i : Inport  Port=4
  Compare To Constant{1..10} (10 alike) : simulink/Logic and Bit Operations/Compare To Constant  relop=>=  const=0  OutDataTypeStr=boolean
  Product{,1..9} (10 alike) : Product
  Sum{1..18,29..30} (20 alike) : Sum  Inputs=++|
  Unit Delay{,1..9} (10 alike) : UnitDelay  SampleTime=-1  HasFrameUpgradeWarning=on
  out_1 : Outport
  L_o : Outport  Port=2
  x_o : Outport  Port=3
  y_o : Outport  Port=4
  wires:
  Sum2/1 -> Sum1/2
  Unit Delay4/1 -> Unit Delay5/1, Product5/2
  Unit Delay9/1 -> x_o/1, Product1/2
  Sum3/1 -> Sum2/2
  Sum6/1 -> Compare To Constant2/1, Sum7/2
  Sum15/1 -> Compare To Constant7/1, Sum16/2
  Sum9/1 -> Sum13/2
  Sum14/1 -> Sum15/2, Compare To Constant6/1
  Compare To Constant4/1 -> Product4/1
  Unit Delay7/1 -> Unit Delay8/1, Product9/2
  Unit Delay6/1 -> Unit Delay7/1, Product8/2
  Sum7/1 -> Compare To Constant3/1, Sum8/2
  Compare To Constant3/1 -> Product3/1
  Product8/1 -> Sum12/1
  Sum13/1 -> Sum12/2
  in_1/1 -> Sum18/1, Sum6/1, Sum7/1, Sum15/1, Sum16/1, out_1/1, Sum30/1, Sum29/1, Sum17/1, Sum14/1, Sum8/1
  Unit Delay8/1 -> Unit Delay9/1, Product6/2
  Product9/1 -> Sum13/1
  Sum11/1 -> Sum10/2
  Sum8/1 -> Compare To Constant4/1, Sum14/2
  Compare To Constant6/1 -> Product5/1
  Product7/1 -> Sum11/1
  Compare To Constant8/1 -> Product8/1
  Product/1 -> Sum1/1
  Unit Delay5/1 -> Unit Delay6/1, Product7/2
  Unit Delay/1 -> Unit Delay1/1, Product/2
  Unit Delay1/1 -> Unit Delay2/1, Product2/2
  Compare To Constant5/1 -> Product6/1
  Sum10/1 -> Sum4/2
  Sum1/1 -> y_o/1
  Compare To Constant2/1 -> Product2/1
  Sum16/1 -> Compare To Constant8/1, Sum17/2
  Compare To Constant1/1 -> Product/1
  Sum4/1 -> Sum3/2
  Sum17/1 -> Sum29/2, Compare To Constant9/1
  Unit Delay3/1 -> Unit Delay4/1, Product4/2
  Product5/1 -> Sum10/1
  Product6/1 -> Sum9/1
  Sum12/1 -> Sum11/2
  Sum29/1 -> Sum30/2, Compare To Constant5/1
  Sum30/1 -> L_o/1, Compare To Constant10/1
  Product4/1 -> Sum4/1
  Product2/1 -> Sum2/1
  Unit Delay2/1 -> Unit Delay3/1, Product3/2
  Compare To Constant9/1 -> Product9/1
  Product3/1 -> Sum3/1
  x_i/1 -> Unit Delay/1
  Compare To Constant7/1 -> Product7/1
  Compare To Constant10/1 -> Product1/1
  Product1/1 -> Sum5/1
  y_i/1 -> Sum5/2
  Sum5/1 -> Sum9/2
  L_i/1 -> Sum18/2
  Sum18/1 -> Compare To Constant1/1, Sum6/2

== system VSD_FD_codegen_V2/VSD_FD_6PH_2N/Subsystem/Element_10_O6 ==
  in_1 : Inport
  L_i : Inport  Port=2
  x_i : Inport  Port=3
  y_i : Inport  Port=4
  Compare To Constant{1..10} (10 alike) : simulink/Logic and Bit Operations/Compare To Constant  relop=>=  const=0  OutDataTypeStr=boolean
  Product{,1..9} (10 alike) : Product
  Sum{1..18,29..30} (20 alike) : Sum  Inputs=++|
  Unit Delay{,1..9} (10 alike) : UnitDelay  SampleTime=-1  HasFrameUpgradeWarning=on
  out_1 : Outport
  L_o : Outport  Port=2
  x_o : Outport  Port=3
  y_o : Outport  Port=4
  wires:
  Sum2/1 -> Sum1/2
  Unit Delay4/1 -> Unit Delay5/1, Product5/2
  Unit Delay9/1 -> x_o/1, Product1/2
  Sum3/1 -> Sum2/2
  Sum6/1 -> Compare To Constant2/1, Sum7/2
  Sum15/1 -> Compare To Constant7/1, Sum16/2
  Sum9/1 -> Sum13/2
  Sum14/1 -> Sum15/2, Compare To Constant6/1
  Compare To Constant4/1 -> Product4/1
  Unit Delay7/1 -> Unit Delay8/1, Product9/2
  Unit Delay6/1 -> Unit Delay7/1, Product8/2
  Sum7/1 -> Compare To Constant3/1, Sum8/2
  Compare To Constant3/1 -> Product3/1
  Product8/1 -> Sum12/1
  Sum13/1 -> Sum12/2
  in_1/1 -> Sum18/1, Sum6/1, Sum7/1, Sum15/1, Sum16/1, out_1/1, Sum30/1, Sum29/1, Sum17/1, Sum14/1, Sum8/1
  Unit Delay8/1 -> Unit Delay9/1, Product6/2
  Product9/1 -> Sum13/1
  Sum11/1 -> Sum10/2
  Sum8/1 -> Compare To Constant4/1, Sum14/2
  Compare To Constant6/1 -> Product5/1
  Product7/1 -> Sum11/1
  Compare To Constant8/1 -> Product8/1
  Product/1 -> Sum1/1
  Unit Delay5/1 -> Unit Delay6/1, Product7/2
  Unit Delay/1 -> Unit Delay1/1, Product/2
  Unit Delay1/1 -> Unit Delay2/1, Product2/2
  Compare To Constant5/1 -> Product6/1
  Sum10/1 -> Sum4/2
  Sum1/1 -> y_o/1
  Compare To Constant2/1 -> Product2/1
  Sum16/1 -> Compare To Constant8/1, Sum17/2
  Compare To Constant1/1 -> Product/1
  Sum4/1 -> Sum3/2
  Sum17/1 -> Sum29/2, Compare To Constant9/1
  Unit Delay3/1 -> Unit Delay4/1, Product4/2
  Product5/1 -> Sum10/1
  Product6/1 -> Sum9/1
  Sum12/1 -> Sum11/2
  Sum29/1 -> Sum30/2, Compare To Constant5/1
  Sum30/1 -> L_o/1, Compare To Constant10/1
  Product4/1 -> Sum4/1
  Product2/1 -> Sum2/1
  Unit Delay2/1 -> Unit Delay3/1, Product3/2
  Compare To Constant9/1 -> Product9/1
  Product3/1 -> Sum3/1
  x_i/1 -> Unit Delay/1
  Compare To Constant7/1 -> Product7/1
  Compare To Constant10/1 -> Product1/1
  Product1/1 -> Sum5/1
  y_i/1 -> Sum5/2
  Sum5/1 -> Sum9/2
  L_i/1 -> Sum18/2
  Sum18/1 -> Compare To Constant1/1, Sum6/2

== system VSD_FD_codegen_V2/VSD_FD_6PH_2N/Subsystem/Element_10_O7 ==
  in_1 : Inport
  L_i : Inport  Port=2
  x_i : Inport  Port=3
  y_i : Inport  Port=4
  Compare To Constant{1..10} (10 alike) : simulink/Logic and Bit Operations/Compare To Constant  relop=>=  const=0  OutDataTypeStr=boolean
  Product{,1..9} (10 alike) : Product
  Sum{1..18,29..30} (20 alike) : Sum  Inputs=++|
  Unit Delay{,1..9} (10 alike) : UnitDelay  SampleTime=-1  HasFrameUpgradeWarning=on
  out_1 : Outport
  L_o : Outport  Port=2
  x_o : Outport  Port=3
  y_o : Outport  Port=4
  wires:
  Sum2/1 -> Sum1/2
  Unit Delay4/1 -> Unit Delay5/1, Product5/2
  Unit Delay9/1 -> x_o/1, Product1/2
  Sum3/1 -> Sum2/2
  Sum6/1 -> Compare To Constant2/1, Sum7/2
  Sum15/1 -> Compare To Constant7/1, Sum16/2
  Sum9/1 -> Sum13/2
  Sum14/1 -> Sum15/2, Compare To Constant6/1
  Compare To Constant4/1 -> Product4/1
  Unit Delay7/1 -> Unit Delay8/1, Product9/2
  Unit Delay6/1 -> Unit Delay7/1, Product8/2
  Sum7/1 -> Compare To Constant3/1, Sum8/2
  Compare To Constant3/1 -> Product3/1
  Product8/1 -> Sum12/1
  Sum13/1 -> Sum12/2
  in_1/1 -> Sum18/1, Sum6/1, Sum7/1, Sum15/1, Sum16/1, out_1/1, Sum30/1, Sum29/1, Sum17/1, Sum14/1, Sum8/1
  Unit Delay8/1 -> Unit Delay9/1, Product6/2
  Product9/1 -> Sum13/1
  Sum11/1 -> Sum10/2
  Sum8/1 -> Compare To Constant4/1, Sum14/2
  Compare To Constant6/1 -> Product5/1
  Product7/1 -> Sum11/1
  Compare To Constant8/1 -> Product8/1
  Product/1 -> Sum1/1
  Unit Delay5/1 -> Unit Delay6/1, Product7/2
  Unit Delay/1 -> Unit Delay1/1, Product/2
  Unit Delay1/1 -> Unit Delay2/1, Product2/2
  Compare To Constant5/1 -> Product6/1
  Sum10/1 -> Sum4/2
  Sum1/1 -> y_o/1
  Compare To Constant2/1 -> Product2/1
  Sum16/1 -> Compare To Constant8/1, Sum17/2
  Compare To Constant1/1 -> Product/1
  Sum4/1 -> Sum3/2
  Sum17/1 -> Sum29/2, Compare To Constant9/1
  Unit Delay3/1 -> Unit Delay4/1, Product4/2
  Product5/1 -> Sum10/1
  Product6/1 -> Sum9/1
  Sum12/1 -> Sum11/2
  Sum29/1 -> Sum30/2, Compare To Constant5/1
  Sum30/1 -> L_o/1, Compare To Constant10/1
  Product4/1 -> Sum4/1
  Product2/1 -> Sum2/1
  Unit Delay2/1 -> Unit Delay3/1, Product3/2
  Compare To Constant9/1 -> Product9/1
  Product3/1 -> Sum3/1
  x_i/1 -> Unit Delay/1
  Compare To Constant7/1 -> Product7/1
  Compare To Constant10/1 -> Product1/1
  Product1/1 -> Sum5/1
  y_i/1 -> Sum5/2
  Sum5/1 -> Sum9/2
  L_i/1 -> Sum18/2
  Sum18/1 -> Compare To Constant1/1, Sum6/2

== system VSD_FD_codegen_V2/VSD_FD_6PH_2N/Subsystem/Element_10_O8 ==
  in_1 : Inport
  L_i : Inport  Port=2
  x_i : Inport  Port=3
  y_i : Inport  Port=4
  Compare To Constant{1..10} (10 alike) : simulink/Logic and Bit Operations/Compare To Constant  relop=>=  const=0  OutDataTypeStr=boolean
  Product{,1..9} (10 alike) : Product
  Sum{1..18,29..30} (20 alike) : Sum  Inputs=++|
  Unit Delay{,1..9} (10 alike) : UnitDelay  SampleTime=-1  HasFrameUpgradeWarning=on
  out_1 : Outport
  L_o : Outport  Port=2
  x_o : Outport  Port=3
  y_o : Outport  Port=4
  wires:
  Sum2/1 -> Sum1/2
  Unit Delay4/1 -> Unit Delay5/1, Product5/2
  Unit Delay9/1 -> x_o/1, Product1/2
  Sum3/1 -> Sum2/2
  Sum6/1 -> Compare To Constant2/1, Sum7/2
  Sum15/1 -> Compare To Constant7/1, Sum16/2
  Sum9/1 -> Sum13/2
  Sum14/1 -> Sum15/2, Compare To Constant6/1
  Compare To Constant4/1 -> Product4/1
  Unit Delay7/1 -> Unit Delay8/1, Product9/2
  Unit Delay6/1 -> Unit Delay7/1, Product8/2
  Sum7/1 -> Compare To Constant3/1, Sum8/2
  Compare To Constant3/1 -> Product3/1
  Product8/1 -> Sum12/1
  Sum13/1 -> Sum12/2
  in_1/1 -> Sum18/1, Sum6/1, Sum7/1, Sum15/1, Sum16/1, out_1/1, Sum30/1, Sum29/1, Sum17/1, Sum14/1, Sum8/1
  Unit Delay8/1 -> Unit Delay9/1, Product6/2
  Product9/1 -> Sum13/1
  Sum11/1 -> Sum10/2
  Sum8/1 -> Compare To Constant4/1, Sum14/2
  Compare To Constant6/1 -> Product5/1
  Product7/1 -> Sum11/1
  Compare To Constant8/1 -> Product8/1
  Product/1 -> Sum1/1
  Unit Delay5/1 -> Unit Delay6/1, Product7/2
  Unit Delay/1 -> Unit Delay1/1, Product/2
  Unit Delay1/1 -> Unit Delay2/1, Product2/2
  Compare To Constant5/1 -> Product6/1
  Sum10/1 -> Sum4/2
  Sum1/1 -> y_o/1
  Compare To Constant2/1 -> Product2/1
  Sum16/1 -> Compare To Constant8/1, Sum17/2
  Compare To Constant1/1 -> Product/1
  Sum4/1 -> Sum3/2
  Sum17/1 -> Sum29/2, Compare To Constant9/1
  Unit Delay3/1 -> Unit Delay4/1, Product4/2
  Product5/1 -> Sum10/1
  Product6/1 -> Sum9/1
  Sum12/1 -> Sum11/2
  Sum29/1 -> Sum30/2, Compare To Constant5/1
  Sum30/1 -> L_o/1, Compare To Constant10/1
  Product4/1 -> Sum4/1
  Product2/1 -> Sum2/1
  Unit Delay2/1 -> Unit Delay3/1, Product3/2
  Compare To Constant9/1 -> Product9/1
  Product3/1 -> Sum3/1
  x_i/1 -> Unit Delay/1
  Compare To Constant7/1 -> Product7/1
  Compare To Constant10/1 -> Product1/1
  Product1/1 -> Sum5/1
  y_i/1 -> Sum5/2
  Sum5/1 -> Sum9/2
  L_i/1 -> Sum18/2
  Sum18/1 -> Compare To Constant1/1, Sum6/2

== system VSD_FD_codegen_V2/VSD_FD_6PH_2N/Subsystem/Element_10_O9 ==
  in_1 : Inport
  L_i : Inport  Port=2
  x_i : Inport  Port=3
  y_i : Inport  Port=4
  Compare To Constant{1..10} (10 alike) : simulink/Logic and Bit Operations/Compare To Constant  relop=>=  const=0  OutDataTypeStr=boolean
  Product{,1..9} (10 alike) : Product
  Sum{1..18,29..30} (20 alike) : Sum  Inputs=++|
  Unit Delay{,1..9} (10 alike) : UnitDelay  SampleTime=-1  HasFrameUpgradeWarning=on
  out_1 : Outport
  L_o : Outport  Port=2
  x_o : Outport  Port=3
  y_o : Outport  Port=4
  wires:
  Sum2/1 -> Sum1/2
  Unit Delay4/1 -> Unit Delay5/1, Product5/2
  Unit Delay9/1 -> x_o/1, Product1/2
  Sum3/1 -> Sum2/2
  Sum6/1 -> Compare To Constant2/1, Sum7/2
  Sum15/1 -> Compare To Constant7/1, Sum16/2
  Sum9/1 -> Sum13/2
  Sum14/1 -> Sum15/2, Compare To Constant6/1
  Compare To Constant4/1 -> Product4/1
  Unit Delay7/1 -> Unit Delay8/1, Product9/2
  Unit Delay6/1 -> Unit Delay7/1, Product8/2
  Sum7/1 -> Compare To Constant3/1, Sum8/2
  Compare To Constant3/1 -> Product3/1
  Product8/1 -> Sum12/1
  Sum13/1 -> Sum12/2
  in_1/1 -> Sum18/1, Sum6/1, Sum7/1, Sum15/1, Sum16/1, out_1/1, Sum30/1, Sum29/1, Sum17/1, Sum14/1, Sum8/1
  Unit Delay8/1 -> Unit Delay9/1, Product6/2
  Product9/1 -> Sum13/1
  Sum11/1 -> Sum10/2
  Sum8/1 -> Compare To Constant4/1, Sum14/2
  Compare To Constant6/1 -> Product5/1
  Product7/1 -> Sum11/1
  Compare To Constant8/1 -> Product8/1
  Product/1 -> Sum1/1
  Unit Delay5/1 -> Unit Delay6/1, Product7/2
  Unit Delay/1 -> Unit Delay1/1, Product/2
  Unit Delay1/1 -> Unit Delay2/1, Product2/2
  Compare To Constant5/1 -> Product6/1
  Sum10/1 -> Sum4/2
  Sum1/1 -> y_o/1
  Compare To Constant2/1 -> Product2/1
  Sum16/1 -> Compare To Constant8/1, Sum17/2
  Compare To Constant1/1 -> Product/1
  Sum4/1 -> Sum3/2
  Sum17/1 -> Sum29/2, Compare To Constant9/1
  Unit Delay3/1 -> Unit Delay4/1, Product4/2
  Product5/1 -> Sum10/1
  Product6/1 -> Sum9/1
  Sum12/1 -> Sum11/2
  Sum29/1 -> Sum30/2, Compare To Constant5/1
  Sum30/1 -> L_o/1, Compare To Constant10/1
  Product4/1 -> Sum4/1
  Product2/1 -> Sum2/1
  Unit Delay2/1 -> Unit Delay3/1, Product3/2
  Compare To Constant9/1 -> Product9/1
  Product3/1 -> Sum3/1
  x_i/1 -> Unit Delay/1
  Compare To Constant7/1 -> Product7/1
  Compare To Constant10/1 -> Product1/1
  Product1/1 -> Sum5/1
  y_i/1 -> Sum5/2
  Sum5/1 -> Sum9/2
  L_i/1 -> Sum18/2
  Sum18/1 -> Compare To Constant1/1, Sum6/2

== matlab function VSD_FD_codegen_V2/Single_Index_Fault_Detection/HystereseBand1 ==
  data: Ri input; Ro output; e input
%Hystereseband, Ausgang Ro ist gleich Ri falls Ri im Bereich von +-e um 1
%ist, ansonsten ist Ro = 0

function Ro = fcn(Ri, e)

% if (1-e <= Ri) & (Ri <= 1+e)      %das funktioniert nicht für einen Vektor
%     Ro = Ri;
% else
%     Ro = 0;
% end

X = ((1-e <= Ri) & (Ri <= 1+e));
Ro = X.*Ri;

== matlab function VSD_FD_codegen_V2/Single_Index_Fault_Detection/Single_Index ==
  data: i_a input; R output; i_b input; i_x input; i_y input; A output; B output
%https://ieeexplore.ieee.org/stamp/stamp.jsp?tp=&arnumber=8948312&tag=1

function [R, A, B]= fcn(i_a, i_b, i_x, i_y)

A= i_x*i_x+i_y*i_y;
B= i_a*i_a+i_b*i_b;


if B == 0
    R=0;
else
    R=A/B;
end

== matlab function VSD_FD_codegen_V2/VSD_FD_6PH_2N/Fehlerindexe_asym_6Ph_2N ==
  data: i_a input; R output; i_b input; i_x input; i_y input; i_z1 input; i_z2 input


%OPF-Fehlerindexe nach Duran: https://ieeexplore.ieee.org/stamp/stamp.jsp?tp=&arnumber=7858758&tag=1

function R = fcn(i_a, i_b, i_x, i_y, i_z1, i_z2)

% bei zwei isolierten Sternpunkten sin i_z1 und i_z2 0 und fallen so aus
% den gleichungen raus, bei einem gemeinsamen Sternpunkt sind sie ungleich
% 0

%%%%% Gleichungen ohne z1, z2
% % Phase a
% R1 = -i_x/(i_a);
% 
% % Phase b
% R2 = i_x/(-i_a+sqrt(3)*i_b-sqrt(3)*i_y);    %sqrt(3) = 1.732050807568877 bringt sowas zu optimieren bei matlab?; 1/sqrt(3)=0.577350269189626
% 
% % Phase c
% R3 = i_x/(-i_a-sqrt(3)*i_b+sqrt(3)*i_y);
% 
% % Phase d
% R4 = i_x/(i_a+1/sqrt(3)*i_b + 1/sqrt(3) * i_y);
% 
% % Phase e
% R5 = i_x/(i_a-1/sqrt(3)*i_b-1/sqrt(3)*i_y);
% 
% % Phase f
% R6 = -i_y/i_b;



% Phase a
R1 = -i_x/(i_a+i_z1);
if isinf(R1) | isnan(R1)
    R1 = 0;
end

% Phase b
R2 = i_x/(-i_a+sqrt(3)*i_b-sqrt(3)*i_y+2*i_z1);   
if isinf(R2) | isnan(R2)
    R2 = 0;
end

% Phase c
R3 = i_x/(-i_a-sqrt(3)*i_b+sqrt(3)*i_y+2*i_z1);
if isinf(R3) | isnan(R3)
    R3 = 0;
end

% Phase d
R4 = i_x/(i_a+1/sqrt(3)*i_b + 1/sqrt(3) * i_y+2/sqrt(3) *i_z2);
if isinf(R4) | isnan(R4)
    R4 = 0;
end

% Phase e
R5 = i_x/(i_a-1/sqrt(3)*i_b-1/sqrt(3)*i_y-2/sqrt(3)*i_z2);
if isinf(R5) | isnan(R5)
    R5 = 0;
end

% Phase f
R6 = -i_y/(i_b-i_z2);
if isinf(R6) | isnan(R6)
    R6 = 0;
end

R=[R1; R2; R3; R4; R5; R6];

== matlab function VSD_FD_codegen_V2/VSD_FD_6PH_2N/HystereseBand ==
  data: Ri input; Ro output; e_u input; e_o input
% Hystereseband, Ausgang Ro ist gleich Ri falls Ri im Bereich von +-e um 1
% ist, ansonsten ist Ro = 0

function Ro = fcn(Ri, e_u, e_o)

% if (1-e <= Ri) & (Ri <= 1+e)      %das funktioniert nicht für einen Vektor
%     Ro = Ri;
% else
%     Ro = 0;
% end

X = ((1-e_u <= Ri) & (Ri <= 1+e_o));
Ro = X.*Ri;

== matlab function VSD_FD_codegen_V2/VSD_FD_6PH_2N/Auswertung ==
  data: e input; F output; th input
function F = fcn(e, th)

F = e > th;

== matlab function VSD_FD_codegen_V2/VSD_FD_6PH_V4/Fehlerindexe_asym_6Ph ==
  data: i_a input; R output; i_b input; i_x input; i_y input; i_z1 input; i_z2 input
%OPF-Fehlerindexe nach Duran: https://ieeexplore.ieee.org/stamp/stamp.jsp?tp=&arnumber=7858758&tag=1

function R = fcn(i_a, i_b, i_x, i_y, i_z1, i_z2)

denum = 0;

% Phase a
denum = (i_a+i_z1);
if denum == 0
    R1 = 0;
else
    R1 = -i_x/denum;
end

% Phase b
denum = (-i_a+sqrt(3)*i_b-sqrt(3)*i_y+2*i_z1);   
if denum == 0
    R2 = 0;
else
    R2 = i_x/denum;
end

% Phase c
denum = (-i_a-sqrt(3)*i_b+sqrt(3)*i_y+2*i_z1);
if denum == 0
    R3 = 0;
else
    R3 = i_x/denum;
end

% Phase d
denum = (i_a+1/sqrt(3)*i_b + 1/sqrt(3) * i_y+2/sqrt(3) *i_z2);
if denum == 0
    R4 = 0;
else
    R4 = i_x/denum;
end

% Phase e
denum = (i_a-1/sqrt(3)*i_b-1/sqrt(3)*i_y-2/sqrt(3)*i_z2);
if denum == 0
    R5 = 0;
else
    R5 = i_x/denum;
end

% Phase f
denum = (i_b-i_z2);
if denum == 0
    R6 = 0;
else
    R6 = -i_y/denum;
end

R=[R1; R2; R3; R4; R5; R6];


% % Phase a
% R1 = -i_x/(i_a+i_z1);
% if isinf(R1) | isnan(R1)
%     R1 = 0;
% end
% 
% % Phase b
% R2 = i_x/(-i_a+sqrt(3)*i_b-sqrt(3)*i_y+2*i_z1);   
% if isinf(R2) | isnan(R2)
%     R2 = 0;
% end
% 
% % Phase c
% R3 = i_x/(-i_a-sqrt(3)*i_b+sqrt(3)*i_y+2*i_z1);
% if isinf(R3) | isnan(R3)
%     R3 = 0;
% end
% 
% % Phase d
% R4 = i_x/(i_a+1/sqrt(3)*i_b + 1/sqrt(3) * i_y+2/sqrt(3) *i_z2);
% if isinf(R4) | isnan(R4)
%     R4 = 0;
% end
% 
% % Phase e
% R5 = i_x/(i_a-1/sqrt(3)*i_b-1/sqrt(3)*i_y-2/sqrt(3)*i_z2);
% if isinf(R5) | isnan(R5)
%     R5 = 0;
% end
% 
% % Phase f
% R6 = -i_y/(i_b-i_z2);
% if isinf(R6) | isnan(R6)
%     R6 = 0;
% end

== matlab function VSD_FD_codegen_V2/VSD_FD_6PH_V4/HystereseBand ==
  data: Ri input; Ro output; e_u input; e_o input
% Hystereseband, Ausgang Ro ist gleich Ri falls Ri im Bereich von +-e um 1
% ist, ansonsten ist Ro = 0

function Ro = fcn(Ri, e_u, e_o)

X = ((1-e_u <= Ri) & (Ri <= 1+e_o));
Ro = X.*Ri;

== matlab function VSD_FD_codegen_V2/VSD_FD_6PH_2N/Auswertung2 ==
  data: e input; F output; th input
function F = fcn(e, th)

F = e > th;

== matlab function VSD_FD_codegen_V2/VSD_FD_6PH_2N/MATLAB Function1 ==
  data: w_el input; N output; f input; k input
% Block zur Bestimmung der Fensterlänge für die Bildung des gleitenden
% Mittelwerts
% Eingänge: w_el: Aktuelle el. Winkelgeschwindigkeit
%           f: Abtastfrequenz der Mittelwertbildung
%           k: Faktor für die Fensterlänge (Mittelwertbildung über k*Periodendauer)
% Ausgänge: N: Fensterlänge/ Anzahl der Abtastwerte über die gemittelt wird


function N = fcn(w_el, f, k)

% finden der aktuellen Periodendauer
w_el = abs(w_el);
T = 2*pi/w_el;

% Anzahl der Abtastwerte pro Periode
N=T*f;
% Anzahl Skalieren und auf ganze Zahl runden
N=k*N;
N= round(N);

% NaN abfangen
if w_el == 0
    N=0;
end

% Begrenzung auf maximale länge
if N > 100
    N = 100;
end

== matlab function VSD_FD_codegen_V2/Single_Index_Fault_Detection/MATLAB Function2 ==
  data: w_el input; N output; f input; k input
% Block zur Bestimmung der Fensterlänge für die Bildung des gleitenden
% Mittelwerts
% Eingänge: w_el: Aktuelle el. Winkelgeschwindigkeit
%           f: Abtastfrequenz der Mittelwertbildung
%           k: Faktor für die Fensterlänge (Mittelwertbildung über k*Periodendauer)
% Ausgänge: N: Fensterlänge/ Anzahl der Abtastwerte über die gemittelt wird


function N = fcn(w_el, f, k)

% finden der aktuellen Periodendauer
w_el = abs(w_el);
T = 2*pi/w_el;

% Anzahl der Abtastwerte pro Periode
N=T*f;
% Anzahl Skalieren und auf ganze Zahl runden
N=k*N;
N= round(N);

% NaN abfangen
if w_el == 0
    N=0;
end

% Begrenzung auf maximale länge
if N > 100
    N = 100;
end
